simulink model "atc_ut"  (Simulink 8.1)
settings: Solver=ode45  StartTime=0.0  StopTime=10.0  RelTol=1e-3
libraries: siltestlib x4, atc x1
settings Model: Creator=AT015086  LastModifiedBy=tescamilla
settings DataIOCC: SignalLoggingSaveFormat=Dataset
settings OptimizationCC: ExpressionDepthLimit=128
settings DebuggingCC: FcnCallInpInsideContextMsg=EnableAllAsError
settings GRTTargetCC: CombineOutputUpdateFcns=on  GRTInterface=off

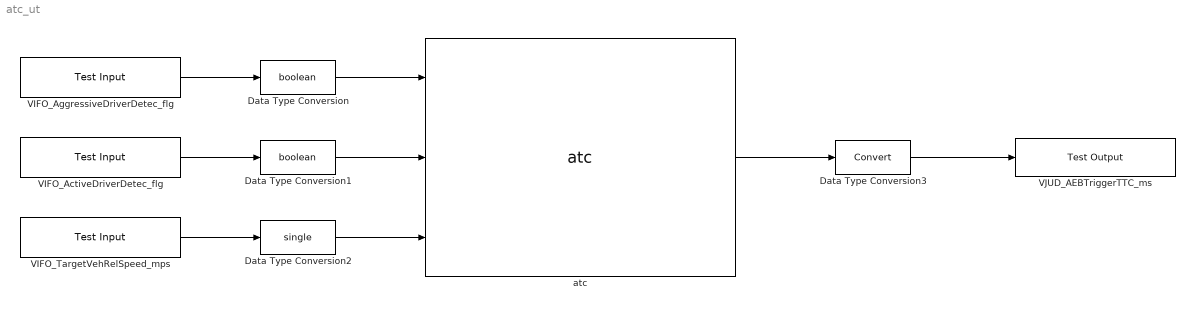
== system atc_ut ==
  Data Type Conversion : DataTypeConversion  OutDataTypeStr=boolean
  Data Type Conversion1 : DataTypeConversion  OutDataTypeStr=boolean
  Data Type Conversion2 : DataTypeConversion  OutDataTypeStr=single
  Data Type Conversion3 : DataTypeConversion
  VIFO_ActiveDriverDetec_flg : siltestlib/Test Input  varname=VIFO_ActiveDriverDetec_flg  sampletime=-1
  VIFO_AggressiveDriverDetec_flg : siltestlib/Test Input  varname=VIFO_AggressiveDriverDetec_flg  sampletime=-1
  VIFO_TargetVehRelSpeed_mps : siltestlib/Test Input  varname=VIFO_TargetVehRelSpeed_mps  sampletime=-1
  VJUD_AEBTriggerTTC_ms : siltestlib/Test Output  varname=VJUD_AEBTriggerTTC_ms  sampletime=-1
  "atc " : atc/atc 
  wires:
  Data Type Conversion/1 -> "atc "/1
  Data Type Conversion1/1 -> "atc "/2
  Data Type Conversion2/1 -> "atc "/3
  "atc "/1 -> Data Type Conversion3/1
  Data Type Conversion3/1 -> VJUD_AEBTriggerTTC_ms/1
  VIFO_AggressiveDriverDetec_flg/1 -> Data Type Conversion/1
  VIFO_ActiveDriverDetec_flg/1 -> Data Type Conversion1/1
  VIFO_TargetVehRelSpeed_mps/1 -> Data Type Conversion2/1
